simulink model "CITRIS_original2"  (Simulink 7.4)
settings: Solver=FixedStepDiscrete  StartTime=0  StopTime=25  FixedStep=1  MaxStep=1  RelTol=1e-3
values from neighbouring files (symbols this model uses):
  mdot = [mdot controlInputHistory{i}(1,:)']    [CITRISBLOMSimulation.m]
  mdotmax = 740    [CITRISBLOMSimulation.m]
  mdotmin = 220    [CITRISBLOMSimulation.m]
  model =     [model.mat]
  vlv = [vlv controlInputHistory{i}(2,:)']    [CITRISBLOMSimulation.m]
undefined symbols (not defined in the file or in its folder): i, mdotTk, mdotvlv, mdotvlvk, Tk, TmaxSlack, TmaxV, TminSlack, TminV, wk, wk_1, wk_2
libraries: MPCMdlLib x19
settings Model: Creator=vichik  LastModifiedBy=Kyle
settings OptimizationCC: InitFltsAndDblsToZero=on

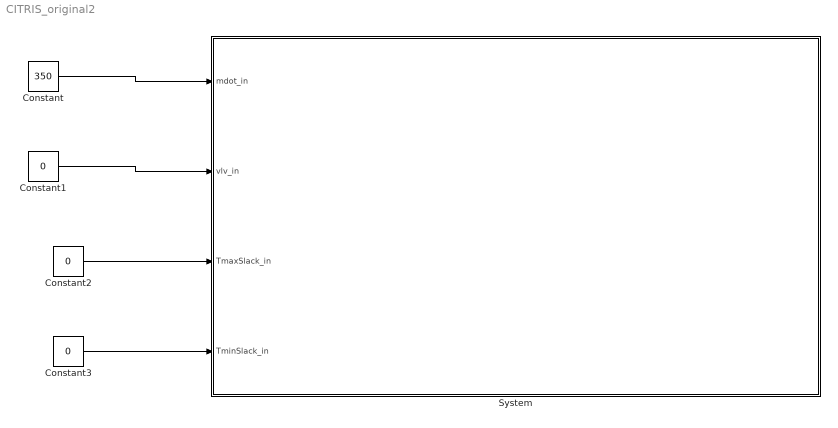
== system CITRIS_original2 ==
  Constant : Constant  Value=350
  Constant1 : Constant  Value=0
  Constant2 : Constant  Value=0
  Constant3 : Constant  Value=0
  System : Subsystem
  wires:
  Constant/1 -> System/1(mdot_in)
  Constant1/1 -> System/2(vlv_in)
  Constant2/1 -> System/3(TmaxSlack_in)
  Constant3/1 -> System/4(TminSlack_in)

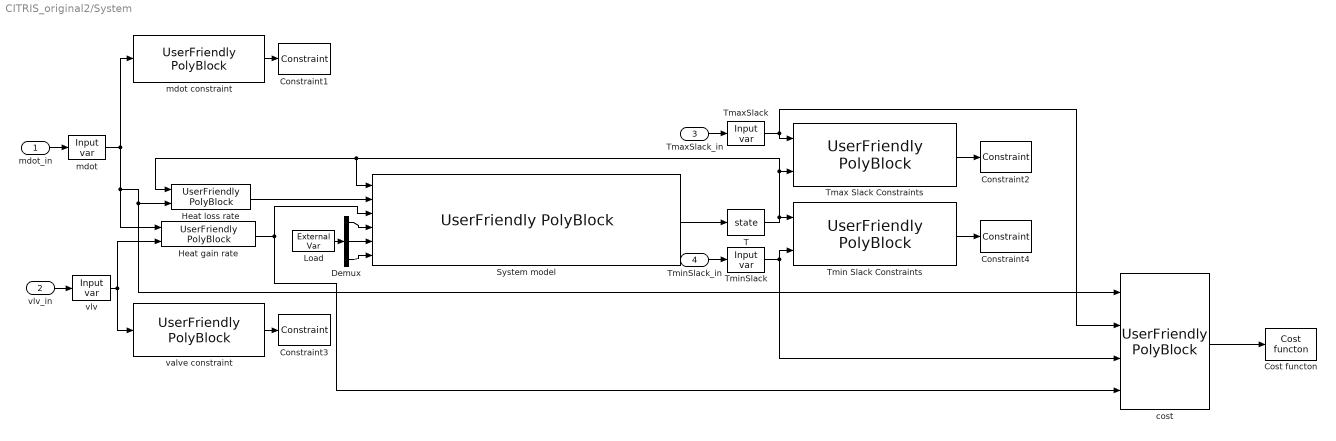
== system CITRIS_original2/System ==
  mdot_in : Inport
  vlv_in : Inport  Port=2
  TmaxSlack_in : Inport  Port=3
  TminSlack_in : Inport  Port=4
  Constraint{1..4} (4 alike) : MPCMdlLib/Constraint  Tag=InequalBlock  CompareSign=< 0
  Cost functon : MPCMdlLib/Cost functon  Tag=OptCost
  Demux : Demux  Outputs=3
  Heat gain rate : MPCMdlLib/UserFriendly PolyBlock  Tag=PolyBlock  A="[1  1  ]"  C=[1 ]  gA=[0 0]  gC=1  input_type=Scalar  output_type=Scalar  port_names=mdot,vlv
  Heat loss rate : MPCMdlLib/UserFriendly PolyBlock  Tag=PolyBlock  A="[1  1  ]"  C=[1 ]  gA=[0 0]  gC=1  input_type=Scalar  output_type=Scalar  port_names=Tk,mdot
  Load : MPCMdlLib/External Var  Tag=OptExternal  SystemSampleTime=-1  step_ratio=1  save_name=BL_System_Load
  System model : MPCMdlLib/UserFriendly PolyBlock  Tag=PolyBlock  A=[1 0 0 0 0 0;0 1 0 0 0 0;0 0 1 0 0 0;0 0 0 1 0 0;0 0 0 0 1 0;0 0 0 0 0 1;0 0 0 0 0 0]  C=[model{i}.A model{i}.B2 model{i}.B1 model{i}.W(1) model{i}.W(2) model{i}.W(3) model{i}.C]  gA=[0 0 0 0 0 0]  gC=1  input_type=Scalar  output_type=Scalar  port_names=Tk,mdotTk,mdotvlvk,wk,wk_1,wk_2
  T : MPCMdlLib/state  Tag=OptState  SystemSampleTime=-1  init_val=T0  save_name=BL_System_T
  Tmax Slack Constraints : MPCMdlLib/UserFriendly PolyBlock  Tag=PolyBlock  A=[0 1;1 0;0 0]  C=[1 -1 -22;0 -1 0]  gA=[0 0]  gC=1  input_type=Scalar  output_type=Vector  port_names=TmaxSlack,Tk
  TmaxSlack : MPCMdlLib/Input var  Tag=OptInput  SystemSampleTime=-1  step_ratio=1  save_name=BL_System_TmaxSlack
  Tmin Slack Constraints : MPCMdlLib/UserFriendly PolyBlock  Tag=PolyBlock  A=[1 0;0 1;0 0]  C=[-1 -1 20;0 -1 0]  gA=[0 0]  gC=1  input_type=Scalar  output_type=Vector  port_names=Tk,TminSlack
  TminSlack : MPCMdlLib/Input var  Tag=OptInput  SystemSampleTime=-1  step_ratio=1  save_name=BL_System_TminSlack
  "cost " : MPCMdlLib/UserFriendly PolyBlock  Tag=PolyBlock  A=[0 0 1 0;0 1 0 0;2 0 0 0;0 0 0 1]  C=[1 1 1e-6 0.01*1e-5]  gA=[0 0 0 0]  gC=1  input_type=Scalar  output_type=Scalar  port_names=mdot,TmaxV,TminV,mdotvlv
  mdot : MPCMdlLib/Input var  Tag=OptInput  SystemSampleTime=-1  step_ratio=1  save_name=BL_System_mdot
  mdot constraint : MPCMdlLib/UserFriendly PolyBlock  Tag=PolyBlock  A="[1  ;  0 ]"  C=[1 -mdotmax; -1 mdotmin]  gA="[0  ]"  gC=1  input_type=Scalar  output_type=Vector  port_names=mdot
  valve constraint : MPCMdlLib/UserFriendly PolyBlock  Tag=PolyBlock  A=[1;0]  C="[1 -100; -1  0]"  gA=[0]  gC=1  input_type=Scalar  output_type=Vector  port_names=vlv
  vlv : MPCMdlLib/Input var  Tag=OptInput  SystemSampleTime=-1  step_ratio=1  save_name=BL_System_vlv
  wires:
  T/1 -> Heat loss rate/1, System model/1, Tmax Slack Constraints/2, Tmin Slack Constraints/1
  mdot/1 -> Heat loss rate/2, "cost "/1, Heat gain rate/1, mdot constraint/1
  "cost "/1 -> Cost functon/1
  mdot_in/1 -> mdot/1
  mdot constraint/1 -> Constraint1/1
  vlv_in/1 -> vlv/1
  vlv/1 -> Heat gain rate/2, valve constraint/1
  valve constraint/1 -> Constraint3/1
  Load/1 -> Demux/1
  Demux/1 -> System model/4
  Demux/2 -> System model/5
  Demux/3 -> System model/6
  Heat loss rate/1 -> System model/2
  Heat gain rate/1 -> System model/3, "cost "/4
  Tmax Slack Constraints/1 -> Constraint2/1
  Tmin Slack Constraints/1 -> Constraint4/1
  TmaxSlack/1 -> "cost "/2, Tmax Slack Constraints/1
  System model/1 -> T/1
  TminSlack/1 -> Tmin Slack Constraints/2, "cost "/3
  TmaxSlack_in/1 -> TmaxSlack/1
  TminSlack_in/1 -> TminSlack/1
